simulink model "promokhaberat"  (R2013a)
settings: Solver=ode45  StartTime=0.0  StopTime=10.0  RelTol=1e-3
settings Model: Creator=engineer  LastModifiedBy=engineer

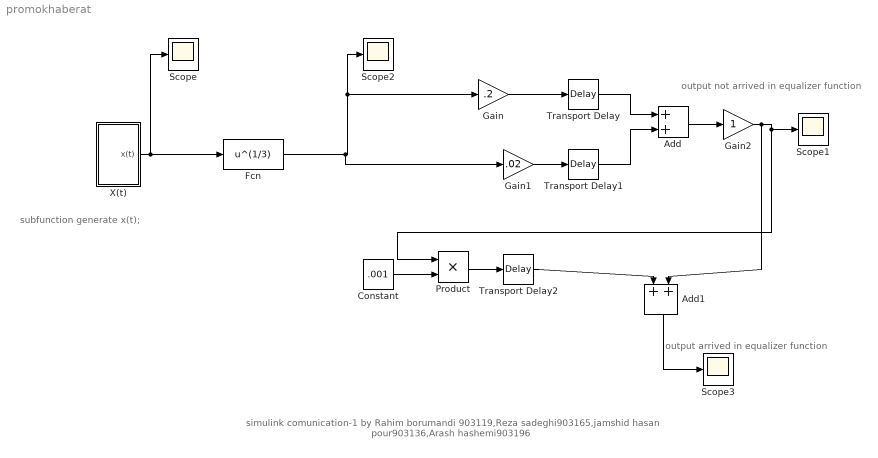
== system promokhaberat ==
  note: output arrived in equalizer function
  note: output not arrived in equalizer function
  note: subfunction generate x(t);
  note: simulink comunication-1 by Rahim borumandi 903119,Reza sadeghi903165,jamshid hasan pour903136,Arash hashemi903196
  Add : Sum
  Add1 : Sum
  Constant : Constant  Value=.001
  Fcn : Fcn  Expr=u^(1/3)
  Gain : Gain  Gain=.2
  Gain1 : Gain  Gain=.02
  Gain2 : Gain
  Product : Product
  Scope{,1..3} (4 alike) : Scope
      Scope2 settings: SaveName=ScopeData5
      Scope3 settings: SaveName=ScopeData6
  Transport Delay : TransportDelay  DelayTime=.5
  Transport Delay1 : TransportDelay  DelayTime=.1
  Transport Delay2 : TransportDelay  DelayTime=.4
  X(t) : Subsystem
  wires:
  Gain1/1 -> Transport Delay1/1
  Gain/1 -> Transport Delay/1
  Transport Delay/1 -> Add/1
  Transport Delay1/1 -> Add/2
  Add/1 -> Gain2/1
  Gain2/1 -> Add1/2, Product/1, Scope1/1
  Fcn/1 -> Gain1/1, Gain/1, Scope2/1
  X(t)/1(x(t)) -> Fcn/1, Scope/1
  Constant/1 -> Product/2
  Product/1 -> Transport Delay2/1
  Transport Delay2/1 -> Add1/1
  Add1/1 -> Scope3/1

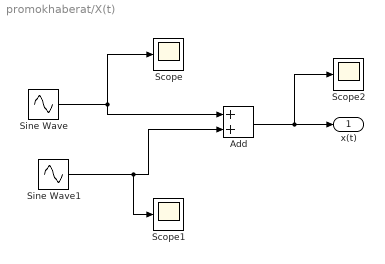
== system promokhaberat/X(t) ==
  Add : Sum
  Scope : Scope
      settings: SaveName=ScopeData2
  Scope1 : Scope
      settings: SaveName=ScopeData3
  Scope2 : Scope
      settings: SaveName=ScopeData4
  Sine Wave : Sin  Amplitude=4  Frequency=126  Phase=pi/2  Samples=1000  SampleTime=0  Offset=100
  Sine Wave1 : Sin  Amplitude=3  Frequency=314  Phase=pi/2  SampleTime=0  Offset=100
  x(t) : Outport
  wires:
  Add/1 -> Scope2/1, x(t)/1
  Sine Wave/1 -> Scope/1, Add/1
  Sine Wave1/1 -> Scope1/1, Add/2
